simulink model "SchemaStavovyOpis"  (R2018b)
settings: Solver=VariableStepAuto  StartTime=0.0  StopTime=10.0  RelTol=1e-3
undefined symbols (not defined in the file): A, B, C, D
settings Model: Creator=Jan  LastModifiedBy=Jan

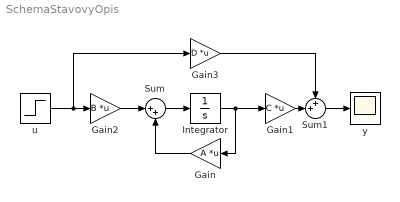
== system SchemaStavovyOpis ==
  Gain : Gain  Gain=A  Multiplication=Matrix(K*u)
  Gain1 : Gain  Gain=C  Multiplication=Matrix(K*u)
  Gain2 : Gain  Gain=B  Multiplication=Matrix(K*u)
  Gain3 : Gain  Gain=D  Multiplication=Matrix(K*u)
  Integrator : Integrator
  Sum : Sum  Inputs=|++
  Sum1 : Sum  Inputs=++|
  u : Step  Time=0  SampleTime=0
  y : Scope
  wires:
  Integrator/1 -> Gain1/1, Gain/1
  Gain/1 -> Sum/2
  Sum/1 -> Integrator/1
  Gain2/1 -> Sum/1
  u/1 -> Gain3/1, Gain2/1
  Gain3/1 -> Sum1/1
  Sum1/1 -> y/1
  Gain1/1 -> Sum1/2
